simulink model "quarc_py_bridge_cp"  (Simulink 8.9)
settings: Solver=ode1  StartTime=0.0  StopTime=inf  FixedStep=0.002  RelTol=1e-3  EnableMultiTasking=on
InitFcn:
  | run('setup_ip02_sip.m')
  | load bus_object_cp.mat
values from neighbouring files (symbols this model uses):
  K_AMP = 1    [setup_ip02_sip.m]
  K_EC = Pr * N_pp / ( 4 * 1024 )    (= 2.27485440932e-05)    [config_ip02.m]
  K_EP = 2 * pi / ( 4 * 1024 )    (= 0.00153398078789)    [config_ip02.m]
  VMAX_DAC = 10    [setup_ip02_sip.m]
undefined symbols (not defined in the file or in its folder): HIL, qc_get_step_size
libraries: quarc_library x5
settings Model: Creator=MLevis  LastModifiedBy=Quanser  SimulationMode=external  ExtModeTrigDuration=5000
settings SolverCC: PositivePriorityOrder=on
settings OptimizationCC: ExpressionDepthLimit=2147483647
settings DebuggingCC: SolverPrmCheckMsg=warning
settings RTWCC: SystemTargetFile=quarc_win64.tlc  TemplateMakefile=quarc_default_tmf  Description=QUARC Win64 Target
settings STFCustomTargetCC: TargetPreCompLibLocation=C:\PROGRA~3\QUARC\lib\2017a\win64\release  ConcurrentExecutionCompliant=on  GeneratePreprocessorConditionals=Disable all  SystemTargetFile=quarc_win64.tlc
settings GRTTargetCC: TargetPreCompLibLocation=C:\PROGRA~3\QUARC\lib\2017a\win64\release  ParMdlRefBuildCompliant=off  CompOptLevelCompliant=off  MatFileLogging=off  CPPClassGenCompliant=off  UseToolchainInfoCompliant=off  ExtMode=on  ExtModeMexFile=quarc_comm
settings ConfigComp: CovSFcnEnable=off

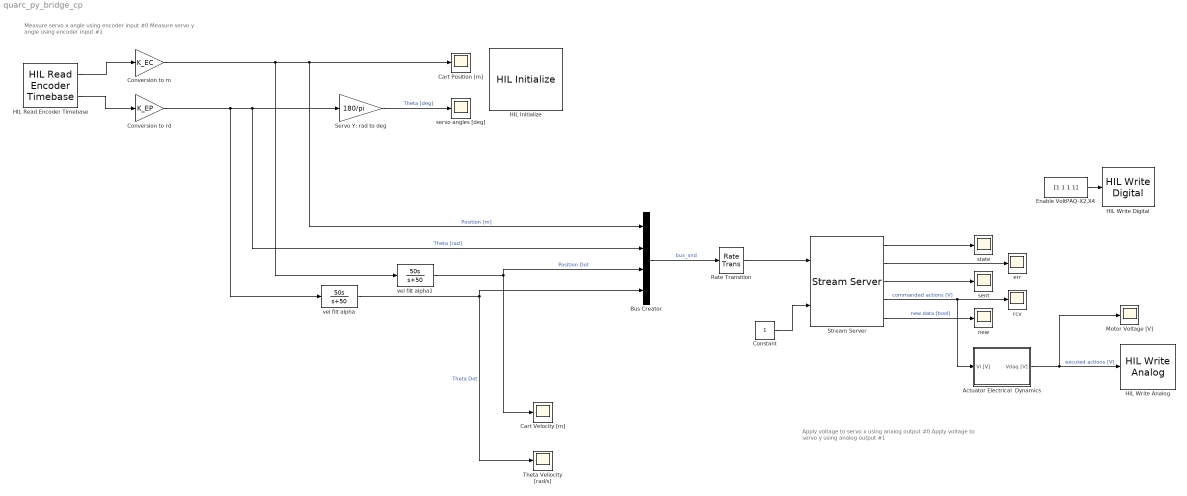
== system quarc_py_bridge_cp ==
  note: Measure servo x angle using encoder input #0
      | Measure servo y angle using encoder input #1
  note: Apply voltage to servo x using analog output #0
      | Apply voltage to servo y using analog output #1
  Actuator Electrical  Dynamics : Subsystem
  Bus Creator : BusCreator  Inputs=4
  "Cart Position [m] " : Scope
  "Cart Velocity [m] " : Scope
  Constant : Constant
  Conversion to m : Gain  Gain=K_EC  SaturateOnIntegerOverflow=on  OutDataTypeStr=Inherit: Same as input  ParamDataTypeStr=Inherit: Same as input
  Conversion to rd : Gain  Gain=K_EP  SaturateOnIntegerOverflow=on  OutDataTypeStr=Inherit: Same as input  ParamDataTypeStr=Inherit: Same as input
  Enable VoltPAQ-X2,X4 : Constant  Value=[1 1 1 1]
  HIL Initialize : quarc_library/Data Acquisition/Generic/Configuration/HIL Initialize  object_name=HIL-1  board_type=q8_usb  board_number=0  board_options=update_rate=normal;decimation=1  exclusive=off  active=on  hardware_clocks=[0:2]  clock_modes=[]  initial_clock_frequencies=[]  set_clock_params_at_start=off  set_clock_params_at_switch_in=off  set_clock_frequencies_at_start=off  set_clock_frequencies_at_switch_in=off  analog_input_channels=[0:7]  analog_input_configurations=[]  analog_input_maximums=10  analog_input_minimums=-10  set_analog_input_params_at_start=on  set_analog_input_params_at_switch_in=off  analog_output_channels=[0:7]  analog_output_maximums=10  analog_output_minimums=-10  initial_analog_outputs=[0]  final_analog_outputs=[0]  watchdog_analog_outputs=0  set_analog_output_params_at_start=on  set_analog_output_params_at_switch_in=off  set_analog_outputs_at_start=on  set_analog_outputs_at_switch_in=off  set_analog_outputs_at_terminate=on  set_analog_outputs_at_switch_out=off  set_analog_outputs_on_watchdog=off  digital_input_channels=[]  digital_output_channels=[0:7]  digital_output_configuration=[]  initial_digital_outputs=[1]  final_digital_outputs=[0]  watchdog_digital_outputs=[0]  set_digital_output_params_at_start=off  set_digital_output_params_at_switch_in=off  set_digital_outputs_at_start=on  set_digital_outputs_at_switch_in=off  set_digital_outputs_at_terminate=on  set_digital_outputs_at_switch_out=off  set_digital_outputs_on_watchdog=off  encoder_channels=[0:7]  quadrature=[4]  encoder_filter_frequency=[]  initial_encoder_counts=[0]  set_encoder_params_at_start=on  set_encoder_params_at_switch_in=off  set_encoder_counts_at_start=on  set_encoder_counts_at_switch_in=off  pwm_channels=[0:7]  pwm_modes=0  pwm_frequency=99.532799999999995e6/4095  pwm_configuration=[0]  pwm_alignment=[0]  pwm_polarity=[1]  pwm_leading_deadband=[0]  pwm_trailing_deadband=[0]  initial_pwm_outputs=[0]  final_pwm_outputs=[0]  watchdog_pwm_outputs=[0]  set_pwm_params_at_start=on  set_pwm_params_at_switch_in=off  set_pwm_outputs_at_start=on  set_pwm_outputs_at_switch_in=off  set_pwm_outputs_at_terminate=on  set_pwm_outputs_at_switch_out=off  set_pwm_outputs_on_watchdog=off  other_output_channels=[]  initial_other_outputs=[]  final_other_outputs=[]  watchdog_other_outputs=[]  set_other_outputs_at_start=off  set_other_outputs_at_switch_in=off  set_other_outputs_at_terminate=off  set_other_outputs_at_switch_out=off  set_other_outputs_on_watchdog=off
      settings: AttributesFormatString=(%<object_name>)
  HIL Read Encoder Timebase : quarc_library/Data Acquisition/Generic/Timebases/HIL Read Encoder Timebase  object_name=HIL-1  clock=0  channels=[0:1]  samples_in_buffer=max(ceil(1/qc_get_step_size), 1)  active=on  vector_output=off  data_type_mode=Inherit via back propagation  data_type=double
  HIL Write Analog : quarc_library/Data Acquisition/Generic/Immediate I//O/HIL Write Analog  Tag=unassigned  object_name=HIL-1  channels=[0]  sample_time=-1  active=off  vector_input=on
  HIL Write Digital : quarc_library/Data Acquisition/Generic/Immediate I//O/HIL Write Digital  object_name=HIL-1  channels=[0:3]  sample_time=-1  active=off  vector_input=on
      settings: SourceProductName=QUARC Targets
  Motor Voltage [V] : Scope
  Rate Transition : RateTransition
  Servo Y: rad to deg : Gain  Gain=180/pi  SaturateOnIntegerOverflow=on  OutDataTypeStr=Inherit: Same as input  ParamDataTypeStr=Inherit: Same as input
  Stream Server : quarc_library/Communications/Basic/Stream Server  uri_source=Specify via dialog (do not evaluate)  uri=tcpip://localhost:9095  apply_uri_to_all_configs=on  send_buffer_size=1460  receive_buffer_size=1460  byte_order=big endian (Motorola - MSB first)  optimization=Minimum latency  send_options=Send most recent data  receive_options=Receive most recent data  default_value=[0]  sample_time=qc_get_step_size * 1  active=off  implementation=Use blocking I/O in a separate thread  send_fifo_size=1000  receive_fifo_size=1000  send_priority=0  receive_priority=0  send_dimensions=off  receive_dimensions=off  max_dimensions=-1  data_type=double  type_expr=BusObject
      settings: AttributesFormatString="\"tcpip://localhost:9095\""
  Theta Veliocity [rad/s] : Scope
  err : Scope
  new : Scope
  rcv : Scope
  sent : Scope
  servo angles [deg] : Scope
  state : Scope
  vel filt alpha : TransferFcn  Numerator=[50 0]  Denominator=[1 50]
  vel filt alpha1 : TransferFcn  Numerator=[50 0]  Denominator=[1 50]
  wires:
  Stream Server/4 -> Actuator Electrical  Dynamics/1(Vi [V]), rcv/1  "commanded actions [V]"
  Stream Server/5 -> new/1  "new data [bool]"
  Stream Server/3 -> sent/1
  Stream Server/1 -> state/1
  Stream Server/2 -> err/1
  Bus Creator/1 -> Rate Transition/1  "bus_snd"
  HIL Read Encoder Timebase/2 -> Conversion to rd/1
  Conversion to m/1 -> Bus Creator/1, "Cart Position [m] "/1, vel filt alpha1/1  "Position [m]"
  Conversion to rd/1 -> vel filt alpha/1, Bus Creator/2, Servo Y: rad to deg/1  "Theta [rad]"
  HIL Read Encoder Timebase/1 -> Conversion to m/1
  Actuator Electrical  Dynamics/1(Vdaq [V]) -> Motor Voltage [V]/1, HIL Write Analog/1  "excuted actions [V]"
  Servo Y: rad to deg/1 -> servo angles [deg]/1  "Theta [deg]"
  Constant/1 -> Stream Server/2
  Enable VoltPAQ-X2,X4/1 -> HIL Write Digital/1
  vel filt alpha/1 -> Theta Veliocity [rad/s]/1, Bus Creator/4  "Theta Dot"
  vel filt alpha1/1 -> "Cart Velocity [m] "/1, Bus Creator/3  "Position Dot"
  Rate Transition/1 -> Stream Server/1

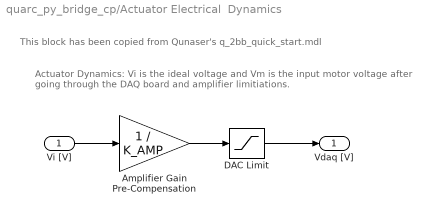
== system quarc_py_bridge_cp/Actuator Electrical  Dynamics ==
  note: Actuator Dynamics: Vi is the ideal voltage and Vm is the
      | input motor voltage after going through the DAQ board and amplifier limitiations.
  note: This block has been copied from Qunaser's q_2bb_quick_start.mdl
  Vi [V] : Inport
  Amplifier Gain Pre-Compensation : Gain  Gain=1 / K_AMP  SaturateOnIntegerOverflow=on  OutDataTypeStr=Inherit: Same as input  ParamDataTypeStr=Inherit: Same as input
  DAC Limit : Saturate  UpperLimit=VMAX_DAC  LowerLimit=- VMAX_DAC
  Vdaq [V] : Outport
  wires:
  Vi [V]/1 -> Amplifier Gain Pre-Compensation/1
  DAC Limit/1 -> Vdaq [V]/1
  Amplifier Gain Pre-Compensation/1 -> DAC Limit/1
